simulink model "simple_charging_stateflow"  (R2024b)
settings: Solver=ode3  StartTime=0.0  StopTime=20.0  FixedStep=1  RelTol=1e-3
libraries: simulink x2
settings Model: Creator=balaj  LastModifiedBy=balaj

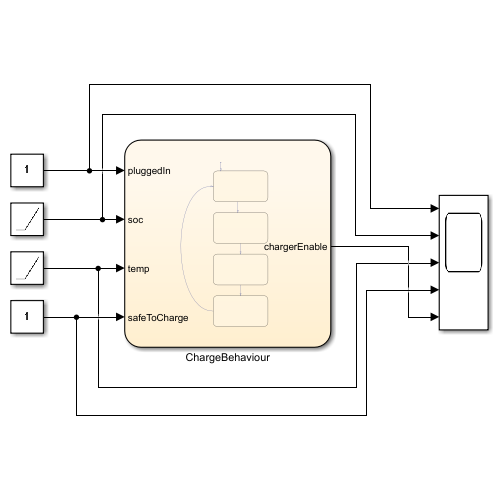
[thumbnail: Simulink's stored preview of the top-level diagram]
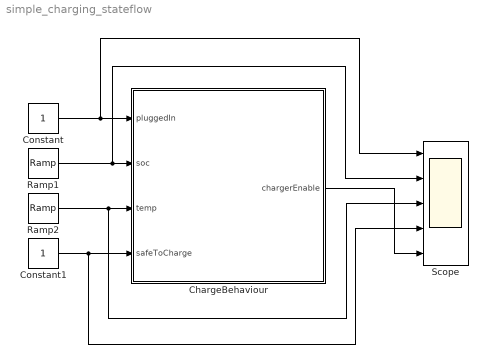
== system simple_charging_stateflow ==
  ChargeBehaviour : Stateflow chart  TreatAsAtomicUnit=on
  Constant : Constant  OutDataTypeStr=boolean
  Constant1 : Constant  OutDataTypeStr=boolean
  Ramp1 : simulink/Sources/Ramp  slope=10  start=0  InitialOutput=0
  Ramp2 : simulink/Sources/Ramp  slope=5  start=0  InitialOutput=0
  Scope : Scope  NumInputPorts=5
  wires:
  Constant/1 -> Scope/1, ChargeBehaviour/1(pluggedIn)
  Ramp1/1 -> Scope/2, ChargeBehaviour/2(soc)
  Ramp2/1 -> Scope/3, ChargeBehaviour/3(temp)
  Constant1/1 -> Scope/4, ChargeBehaviour/4(safeToCharge)
  ChargeBehaviour/1(chargerEnable) -> Scope/5

== stateflow chart simple_charging_stateflow/ChargeBehaviour ==
  state Idle
    entry:
    chargerEnable=0;
  state PreCharge
    entry:
    chargerEnable=0;
  state Charging
    entry:
    chargerEnable=1;
  state Cutoff
    entry:
    chargerEnable=0;
  (default) -> Idle
  Cutoff -> Idle : [pluggedIn==0]
  Idle -> PreCharge : [pluggedIn==1]
  PreCharge -> Charging : [safeToCharge==1]
  Charging -> Cutoff : [soc>=95 || temp>=45]
  data: pluggedIn input boolean; soc input double; temp input double; safeToCharge input boolean; chargerEnable output
